simulink library "BMSInputProcessing"  (R2025a)
settings: Solver=VariableStepAuto  StartTime=0.0  StopTime=10.0  RelTol=1e-3
undefined symbols (not defined in the file or in its folder): raptor_xcp_function, StateCAN
libraries: Utilities x181, Raptor_lib x65, simulink x1
(part 1 of 2)
settings Model: Creator=hyuga  LastModifiedBy=hyuga

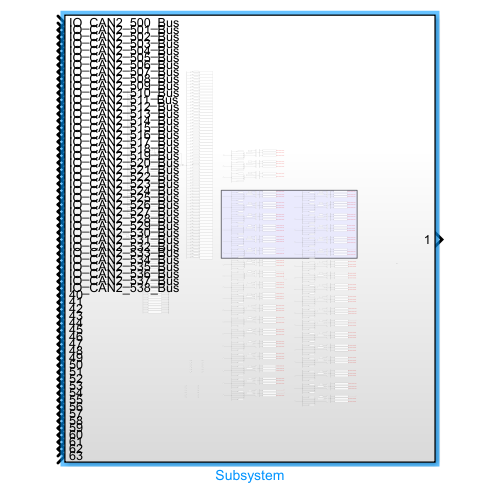
[thumbnail: Simulink's stored preview of the top-level diagram]
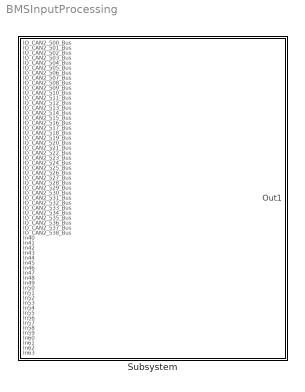
== system BMSInputProcessing ==
  Subsystem : Subsystem
